simulink model "ACC_speed_change_curve_cs"  (R2016a)
settings: Solver=ode5  SolverMode=SingleTasking  StartTime=0.0  StopTime=inf  FixedStep=1/1000  RelTol=1e-3
PreLoadFcn:
  | mbxruntime.callbacks.PreLoadFcn(bdroot);
  | check_NUTS_defined;
  | 
  | assignin('base',['model_closed_' bdroot],false);addpath('../includes_ACC');
PostLoadFcn:
  | mbxruntime.callbacks.PostLoadFcn(bdroot);
InitFcn:
  | mbxruntime.callbacks.InitFcn(bdroot);
StartFcn:
  | mbxruntime.callbacks.StartFcn(bdroot);
StopFcn:
  | mbxruntime.callbacks.StopFcn(bdroot);
model workspace (MAT data in the model file):
  mbox_table : struct (value not decoded)
  model_closed = 0
  sim_status = 0
undefined symbols (not defined in the file or in its folder): DiscIntNeverNeededParam
undefined symbols (not defined in the file): SteeringColumn, SteeringWheel, WheelL0, WheelL1, WheelR0, WheelR1
libraries: simulink_extras x49, simulink x29, PreScanSimulinkLibrary x24, PreScanUsefulBlocks x2, Solver_SF x1, simulink_need_slupdate x1
(part 15 of 17)

== system ACC_speed_change_curve_cs/Audi_A8_1/ACC_System/TIS2 Straight Road/TIS2 Lead Car Longitudinal Velocity ==
  note: === TIS2 Lead Car Longitudinal Velocity block ===
      |
      |  - computes the leading car absolute velocity and safe distance between the EGO and leading car.
  HWT_dem (s) : Inport
  TIS2 Rangedot [m/s] : Inport  Port=2
  EGO Velocity [m/s] : Inport  Port=3
  Standstill [m] : Inport  Port=4
  Abs : Abs
  Add : Sum  Inputs=+-
  Constant : Constant  Value=0
  Divide : Product  Inputs=*/
  HWT_dem (s)1 : InportShadow
  Product : Product  RndMeth=Zero
  Relational Operator : RelationalOperator  Operator=<=  OutDataTypeStr=boolean
  Switch : Switch  Criteria=u2 > Threshold
  Switch1 : Switch  Criteria=u2 ~= 0
  TIS2 Rangedot [m/s]1 : InportShadow  Port=2
  Safe distance [m] : Outport
  Lead velocity [m/s] : Outport  Port=2
  wires:
  Relational Operator/1 -> Switch/2
  Divide/1 -> Relational Operator/2
  HWT_dem (s)1/1 -> Divide/2
  Standstill [m]/1 -> Switch/1, Divide/1
  Switch/1 -> Safe distance [m]/1
  Product/1 -> Switch/3
  HWT_dem (s)/1 -> Product/2
  Add/1 -> Abs/1
  TIS2 Rangedot [m/s]/1 -> Add/2
  EGO Velocity [m/s]/1 -> Add/1
  Constant/1 -> Switch1/3
  Switch1/1 -> Lead velocity [m/s]/1
  TIS2 Rangedot [m/s]1/1 -> Switch1/2
  Abs/1 -> Product/1, Relational Operator/1, Switch1/1

== system ACC_speed_change_curve_cs/Audi_A8_1/ACC_System/TIS2 Straight Road/TIS2 Objects On Lane ==
  note: === TIS2 Objects On Lane block ===
      |
      |  - decides which objects are on the same lane as the EGO car,
      |    when the EGO car drives straight.
  TIS2_range [m] : Inport
  TIS2_rangedot [m/s] : Inport  Port=2
  TIS2_theta [rad] : Inport  Port=3
  Abs : Abs
  Compare To Constant : simulink/Logic and Bit Operations/Compare To Constant  relop=<  const=LaneWidth/2  OutDataTypeStr=boolean
  Constant : Constant  Value=0
  Product : Product  RndMeth=Zero
  Product1 : Product  RndMeth=Zero
  Switch1 : Switch  Criteria=u2 > Threshold  Threshold=0.5
  Switch3 : Switch  Criteria=u2 > Threshold  Threshold=0.5
  TIS2 range max (higher value) : Constant  Value=5*TISMaxRange(2)
  Trigonometric Function : Trigonometry
  Trigonometric Function1 : Trigonometry  Operator=cos
  TIS2_RANGEDOT [m/s] : Outport
  TIS2_Distance [m] : Outport  Port=2
  wires:
  Compare To Constant/1 -> Switch1/2, Switch3/2
  Constant/1 -> Switch1/3
  TIS2 range max (higher value)/1 -> Switch3/3
  Product1/1 -> Switch3/1
  Trigonometric Function1/1 -> Product1/2
  Abs/1 -> Trigonometric Function/1
  Switch3/1 -> TIS2_Distance [m]/1
  Switch1/1 -> TIS2_RANGEDOT [m/s]/1
  TIS2_rangedot [m/s]/1 -> Switch1/1
  TIS2_range [m]/1 -> Product/1, Product1/1
  Product/1 -> Compare To Constant/1
  Trigonometric Function/1 -> Product/2
  TIS2_theta [rad]/1 -> Trigonometric Function1/1, Abs/1

== system ACC_speed_change_curve_cs/Audi_A8_1/ACC_System/TIS2 Straight Road/TIS2 Sorting Fun ==
  note: === TIS2 Sorting Fun block ===
      |
      |  - transforms information from the second sensor
      |    to the more appropriate form.
  TIS2range [m] : Inport
  TIS2rangedot [m/s] : Inport  Port=2
  TIS2theta [deg] : Inport  Port=3
  Degrees to Radians : simulink_extras/Transformations/Degrees to Radians
  Switch : Switch  Criteria=u2 ~= 0
  Unary Minus : UnaryMinus
  Unary Minus1 : UnaryMinus
  range max (higher value which will not generate high level of HWT flag) : Constant  Value=5*TISMaxRange(2)
  TIS2_RANGE [m] : Outport
  TIS2_RANGEDOT [m/s] : Outport  Port=2
  TIS2_THETA [rad] : Outport  Port=3
  wires:
  Unary Minus1/1 -> TIS2_RANGEDOT [m/s]/1
  TIS2theta [deg]/1 -> Unary Minus/1
  TIS2range [m]/1 -> Switch/2, Switch/1
  Degrees to Radians/1 -> TIS2_THETA [rad]/1
  range max (higher value which will not generate high level of HWT flag)/1 -> Switch/3
  TIS2rangedot [m/s]/1 -> Unary Minus1/1
  Switch/1 -> TIS2_RANGE [m]/1
  Unary Minus/1 -> Degrees to Radians/1

== system ACC_speed_change_curve_cs/Audi_A8_1/ACC_System3/Display/If Action Subsystem ==
  note: === Display Module ===
      |
      |  - calls a GUI, which is updated at each step time,
      |  - Inputs for 'DISPLAY' block (msfcn_PlotSpeed):
      |    1 - RPM
      |    2 - EGO Velocity [kph]
      |    3 - Brake Pressure [bar]
      |    4 - Throttle [%]
      |    5 - ACC Flag
      |    6 - HWT converted
      |    7 - Lead car velocity [m/s]
      |
      |  - Output from DISPLAY block (msfcn_ACC_PlotSpeed function):
      |    1 - ACC system manual switch {0 - system off, 1 - system on}
  RPM1 : Inport
  EGO Velocity [m/s]1 : Inport  Port=2
  Brake_Pressure_[bar]1 : Inport  Port=3
  HWT_%1 : Inport  Port=4
  ACC_flag1 : Inport  Port=5
  Lead_car_velocity_[m/s]1 : Inport  Port=6
  Throttle_[%]1 : Inport  Port=7
  Action Port : ActionPort  PropagateVarSize=During execution  ActionType=then
  Brake Pressure [bar] : Gain  Gain=100/BrakePressureMax
  Brake Pressure [bar]1 : Gain  Gain=3.6
  DISPLAY : M-S-Function  FunctionName=msfcn_ACC_PlotSpeed  Parameters=DisplayFreq DisplaySwitch
      mask Display:
      | port_label('input',1,'RPM');
      | port_label('input',2,'EGO Velocity [km/h]');
      | port_label('input',3,'Brake Pressure [bar]');
      | port_label('input',4,'Throttle [%]');
      | port_label('input',5,'ACC Flag');
      | port_label('input',6,'HWT/HWT_dem-1 [%]');
      | port_label('input',7,'Lead car velocity [m/s]');
      | 
      | port_label('output',1,'System On/Off');
  Gain : Gain  OutDataTypeStr=double
  Rounding Function{,1..4,6} (6 alike) : Rounding  Operator=round
  m/s_kph1 : Gain  Gain=3.6
  "GUI_System ON {1} / OFF {0}1" : Outport  InitialOutput=1
  wires:
  Brake Pressure [bar]1/1 -> Rounding Function1/1
  HWT_%1/1 -> DISPLAY/6
  DISPLAY/1 -> "GUI_System ON {1} / OFF {0}1"/1
  Lead_car_velocity_[m/s]1/1 -> m/s_kph1/1
  ACC_flag1/1 -> Gain/1
  EGO Velocity [m/s]1/1 -> Brake Pressure [bar]1/1
  Gain/1 -> Rounding Function6/1
  Rounding Function6/1 -> DISPLAY/5
  Rounding Function4/1 -> DISPLAY/7
  m/s_kph1/1 -> Rounding Function4/1
  RPM1/1 -> Rounding Function/1
  Throttle_[%]1/1 -> Rounding Function3/1
  Brake_Pressure_[bar]1/1 -> Brake Pressure [bar]/1
  Brake Pressure [bar]/1 -> Rounding Function2/1
  Rounding Function3/1 -> DISPLAY/4
  Rounding Function2/1 -> DISPLAY/3
  Rounding Function1/1 -> DISPLAY/2
  Rounding Function/1 -> DISPLAY/1

== system ACC_speed_change_curve_cs/Audi_A8_1/ACC_System3/Display/If Action Subsystem1 ==
  Action Port : ActionPort  PropagateVarSize=During execution  ActionType=else
  Constant : Constant
  Out1 : Outport  InitialOutput=1
  wires:
  Constant/1 -> Out1/1

== system ACC_speed_change_curve_cs/Audi_A8_1/ACC_System3/Limitations1/cond ==
  In1 : Inport
  Integer Delay : Delay  DelayLength=1/Tsensor  InputProcessing=Inherited  SampleTime=Tsensor
  Logical Operator2 : Logic  Operator=NOT  AllPortsSameDT=off  OutDataTypeStr=boolean
  Logical Operator3 : Logic  Operator=OR  AllPortsSameDT=off  OutDataTypeStr=boolean
  Out1 : Outport
  wires:
  Logical Operator3/1 -> Out1/1
  In1/1 -> Logical Operator2/1
  Integer Delay/1 -> Logical Operator3/2
  Logical Operator2/1 -> Integer Delay/1, Logical Operator3/1

== system ACC_speed_change_curve_cs/Audi_A8_1/ACC_System3/Limitations2/cond1 ==
  In1 : Inport
  Integer Delay : Delay  DelayLength=1/Tsensor  InputProcessing=Inherited  SampleTime=Tsensor
  Logical Operator3 : Logic  Operator=OR  AllPortsSameDT=off  OutDataTypeStr=boolean
  Out1 : Outport
  wires:
  Logical Operator3/1 -> Out1/1
  In1/1 -> Integer Delay/1, Logical Operator3/1
  Integer Delay/1 -> Logical Operator3/2

== system ACC_speed_change_curve_cs/Audi_A8_1/ACC_System3/Radar/Radar ==
  TIS1 Range : Inport
  TIS1 Theta : Inport  Port=2
  TIS2 Range : Inport  Port=3
  TIS2 Theta : Inport  Port=4
  TIS1_index : Inport  Port=5
  TIS2_index : Inport  Port=6
  TIS1_HWT_% : Inport  Port=7
  TIS2_HWT_% : Inport  Port=8
  System switch : Inport  Port=9
  Enable : EnablePort  PropagateVarSize=During execution
  Level-2 M-file S-Function : M-S-Function  FunctionName=msfcn_ACC_radar_graph  Parameters=RadarFreq TISdet TISMaxRange TISMaxTheta RadarSwitch
  Logical Operator : Logic  AllPortsSameDT=off  OutDataTypeStr=boolean
  Logical Operator1 : Logic  AllPortsSameDT=off  OutDataTypeStr=boolean
  Product1 : Product  RndMeth=Zero
  Product2 : Product  RndMeth=Zero
  wires:
  TIS2_index/1 -> Product2/1
  TIS1_index/1 -> Product1/1
  Product1/1 -> Level-2 M-file S-Function/5
  Product2/1 -> Level-2 M-file S-Function/6
  System switch/1 -> Product1/2, Product2/2, Logical Operator/2, Logical Operator1/2
  Logical Operator1/1 -> Level-2 M-file S-Function/8
  Logical Operator/1 -> Level-2 M-file S-Function/7
  TIS2_HWT_%/1 -> Logical Operator1/1
  TIS1_HWT_%/1 -> Logical Operator/1
  TIS2 Theta/1 -> Level-2 M-file S-Function/4
  TIS2 Range/1 -> Level-2 M-file S-Function/3
  TIS1 Theta/1 -> Level-2 M-file S-Function/2
  TIS1 Range/1 -> Level-2 M-file S-Function/1

== system ACC_speed_change_curve_cs/Audi_A8_1/ACC_System3/TIS1 ACC action/If Action Subsystem ==
  rd : Inport
  e : Inport  Port=2
  Vp : Inport  Port=3
  EGO distance : Inport  Port=4
  HWT dem : Inport  Port=5
  th in : Inport  Port=6
  Action Port : ActionPort  PropagateVarSize=During execution  ActionType=then
  If : If  IfExpression=u1 <= 0  SampleTime=Tsensor
  If Action Subsystem : Subsystem  TreatAsAtomicUnit=on
  If Action Subsystem1 : Subsystem  TreatAsAtomicUnit=on
  Merge : Merge
  Merge1 : Merge
  Rate Limiter : RateLimiter  RisingSlewLimit=BrakeMax*1e3  FallingSlewLimit=-BrakeMax*1e3  SampleTimeMode=inherited
  e1 : InportShadow  Port=2
  th in1 : InportShadow  Port=6
  dec : Outport  InitialOutput=0
  throttle : Outport  Port=2  InitialOutput=0
  wires:
  Rate Limiter/1 -> throttle/1
  th in1/1 -> If Action Subsystem1/6(th_in)
  th in/1 -> If Action Subsystem/2(th_in)
  HWT dem/1 -> If Action Subsystem1/5(HWT_dem)
  EGO distance/1 -> If Action Subsystem1/4(EGO distance)
  e1/1 -> If Action Subsystem1/2(e)
  Vp/1 -> If Action Subsystem1/3(Vp)
  Merge1/1 -> Rate Limiter/1
  Merge/1 -> dec/1
  If Action Subsystem1/2(throttle) -> Merge1/2
  If Action Subsystem/2(throttle) -> Merge1/1
  If Action Subsystem1/1(dec) -> Merge/2
  If Action Subsystem/1(brake) -> Merge/1
  e/1 -> If Action Subsystem/1(e)
  If/2 -> If Action Subsystem1/Action
  If/1 -> If Action Subsystem/Action
  rd/1 -> If Action Subsystem1/1(rd), If/1

== system ACC_speed_change_curve_cs/Audi_A8_1/ACC_System3/TIS1 ACC action/If Action Subsystem1 ==
  rd : Inport
  e : Inport  Port=2
  Vp : Inport  Port=3
  EGO dis : Inport  Port=4
  HWT dem : Inport  Port=5
  Action Port : ActionPort  PropagateVarSize=During execution  ActionType=else
  If : If  IfExpression=u1 <= 0  SampleTime=Tsensor
  If Action Subsystem : Subsystem  TreatAsAtomicUnit=on
  If Action Subsystem1 : Subsystem  TreatAsAtomicUnit=on
  Merge : Merge
  Merge1 : Merge
  dec : Outport  InitialOutput=0
  throttle : Outport  Port=2  InitialOutput=0
  wires:
  HWT dem/1 -> If Action Subsystem1/5(HWT dem)
  EGO dis/1 -> If Action Subsystem1/4(Ego distance)
  e/1 -> If Action Subsystem1/2(e)
  If Action Subsystem/2(throttle) -> Merge1/1
  If Action Subsystem1/1(dec) -> Merge/2
  Merge1/1 -> throttle/1
  Merge/1 -> dec/1
  If Action Subsystem1/2(throttle) -> Merge1/2
  If Action Subsystem/1(dec) -> Merge/1
  Vp/1 -> If Action Subsystem1/3(Vp)
  If/2 -> If Action Subsystem1/Action
  If/1 -> If Action Subsystem/Action
  rd/1 -> If Action Subsystem1/1(rd), If/1

== system ACC_speed_change_curve_cs/Audi_A8_1/ACC_System3/TIS1 Bend Road/Hold ==
  HWTflagIN : Inport
  lead_vel_in : Inport  Port=2
  HWTflagIN1 : InportShadow
  If : If  IfExpression=u1 < 0.1  SampleTime=Tsensor
  If Action Subsystem : Subsystem  TreatAsAtomicUnit=on
  If Action Subsystem1 : Subsystem  TreatAsAtomicUnit=on
  Merge : Merge
  HWT_flag : Outport
  wires:
  HWTflagIN1/1 -> If Action Subsystem/1(In1)
  HWTflagIN/1 -> If Action Subsystem1/1(In1)
  Merge/1 -> HWT_flag/1
  If Action Subsystem1/1(Out1) -> Merge/2
  If Action Subsystem/1(Out1) -> Merge/1
  If/2 -> If Action Subsystem1/Action
  If/1 -> If Action Subsystem/Action
  lead_vel_in/1 -> If/1

== system ACC_speed_change_curve_cs/Audi_A8_1/ACC_System3/TIS1 Bend Road/Lead Car Longitudinal Velocity ==
  note: === TIS1 Lead Car Longitudinal Velocity block ===
      |
      |  - computes the leading car absolute velocity and safe distance between the EGO and leading car.
  HWT_dem (s) : Inport
  TIS1 Rangedot [m/s] : Inport  Port=2
  EGO Velocity [m/s] : Inport  Port=3
  Standstill [m] : Inport  Port=4
  theta [rad] : Inport  Port=5
  lambda [rad] : Inport  Port=6
  TIS1 Range [m] : Inport  Port=7
  Abs : Abs
  Add : Sum  Inputs=+-  RndMeth=Zero
  Add1 : Sum  Inputs=+-
  Constant : Constant  Value=0
  Divide : Product  Inputs=*/
  Divide2 : Product  Inputs=*/
  HWT_dem (s)1 : InportShadow
  Product : Product  RndMeth=Zero
  Relational Operator : RelationalOperator  Operator=<=  OutDataTypeStr=boolean
  Switch : Switch  Criteria=u2 > Threshold
  Switch1 : Switch  Threshold=TISMaxRange(1)
  Trigonometric Function : Trigonometry  Operator=cos
  Safe distance [m] : Outport
  Lead velocity [m/s] : Outport  Port=2
  wires:
  Switch1/1 -> Lead velocity [m/s]/1
  Constant/1 -> Switch1/1
  TIS1 Range [m]/1 -> Switch1/2
  Abs/1 -> Switch1/3, Relational Operator/1, Product/1
  Divide2/1 -> Add/2
  Trigonometric Function/1 -> Divide2/2
  Add1/1 -> Trigonometric Function/1
  theta [rad]/1 -> Add1/2
  lambda [rad]/1 -> Add1/1
  EGO Velocity [m/s]/1 -> Add/1
  TIS1 Rangedot [m/s]/1 -> Divide2/1
  Add/1 -> Abs/1
  HWT_dem (s)/1 -> Product/2
  Product/1 -> Switch/3
  Switch/1 -> Safe distance [m]/1
  Standstill [m]/1 -> Divide/1, Switch/1
  HWT_dem (s)1/1 -> Divide/2
  Divide/1 -> Relational Operator/2
  Relational Operator/1 -> Switch/2

== system ACC_speed_change_curve_cs/Audi_A8_1/ACC_System3/TIS1 Bend Road/TIS1 Closest Object On Bend Road ==
  note: === TIS1 Closest Object block ===
      |
      |  - passing through data about potentially the most dangerous object driving on the bend road.
  index : Inport
  TIS1_range [m] : Inport  Port=2
  TIS1_rangedot [m] : Inport  Port=3
  TIS1_theta [rad] : Inport  Port=4
  TIS1_Distance [m] : Inport  Port=5
  TIS1_lambda [rad] : Inport  Port=6
  Constant2 : Constant  Value=TISMaxRange(1)
  Selector{1..3,6..7} (5 alike) : Selector  InputPortWidth=TISdet(1)  IndexOptions=Index vector (port)  Indices=[1 3]  OutputSizes=1
  Switch : Switch  Criteria=u2 ~= 0
  range [m] : Outport
  rangedot [m/s] : Outport  Port=2
  theta [rad] : Outport  Port=3
  Distance [m] : Outport  Port=4
  lambda [rad] : Outport  Port=5
  wires:
  Switch/1 -> Distance [m]/1
  Constant2/1 -> Switch/3
  Selector6/1 -> Switch/1, Switch/2
  Selector7/1 -> lambda [rad]/1
  Selector3/1 -> theta [rad]/1
  Selector2/1 -> rangedot [m/s]/1
  Selector1/1 -> range [m]/1
  TIS1_lambda [rad]/1 -> Selector7/1
  TIS1_Distance [m]/1 -> Selector6/1
  TIS1_theta [rad]/1 -> Selector3/1
  index/1 -> Selector7/2, Selector6/2, Selector3/2, Selector2/2, Selector1/2
  TIS1_range [m]/1 -> Selector1/1
  TIS1_rangedot [m]/1 -> Selector2/1

== system ACC_speed_change_curve_cs/Audi_A8_1/ACC_System3/TIS1 Bend Road/TIS1 HWT Computing ==
  note: === TIS1 HWT Computing block===
      |
      |  - computes HeadWay Time (HWT) as it is defined in ISO norms.
  Distance [m] : Inport
  Velocity [m/s] : Inport  Port=2
  If : If
  If Action Subsystem : Subsystem  TreatAsAtomicUnit=on
  If Action Subsystem1 : Subsystem  TreatAsAtomicUnit=on
  Merge : Merge
  HWT [s] : Outport
  wires:
  Distance [m]/1 -> If Action Subsystem/1(Distance [m])
  Merge/1 -> HWT [s]/1
  If Action Subsystem1/1(Out1) -> Merge/2
  If Action Subsystem/1(HWT [s]) -> Merge/1
  If/2 -> If Action Subsystem1/Action
  If/1 -> If Action Subsystem/Action
  Velocity [m/s]/1 -> If Action Subsystem/2(Velocity [m/s]), If/1

== system ACC_speed_change_curve_cs/Audi_A8_1/ACC_System3/TIS1 Bend Road/TIS1 HWT Flag ==
  note: === TIS1 HWT Flag block ===
      |
      |  - outputs the HeadWay Time (HWT) flag,
      |  - holds a high level if the criteria were met,
      |  - sets HWT flag to low level if leading car
      |    went outside the scope of the sensors.
  Distance closest [m] : Inport
  HWT [s] : Inport  Port=2
  HWT_dem [s] : Inport  Port=3
  Standstill distance : Inport  Port=4
  Abs : Abs
  Compare To Constant1 : simulink/Logic and Bit Operations/Compare To Constant  relop===  const=TISMaxRange(1)  OutDataTypeStr=uint8
  Constant : Constant
  Constant1 : Constant  Value=0
  Data Type Conversion : DataTypeConversion
  Data Type Conversion1 : DataTypeConversion
  Discrete-Time Integrator : DiscreteIntegrator  ExternalReset=level  SampleTime=Tsensor  ICPrevOutput=DiscIntNeverNeededParam  ICPrevScaledInput=DiscIntNeverNeededParam
  Distance closest [m]1 : InportShadow
  Gain : Gain  Gain=2
  Gain1 : Gain
  Gain2 : Gain  Gain=1e6  OutDataTypeStr=double
  Gain3 : Gain  Gain=1e6  OutDataTypeStr=double
  Gain4 : Gain  Gain=1.25
  Gain6 : Gain  Gain=100
  Gain7 : Gain  Gain=1.25
  Gain8 : Gain  Gain=0.01
  HWT [s]1 : InportShadow  Port=2
  HWT [s]2 : InportShadow  Port=2
  HWT_dem [s]1 : InportShadow  Port=3
  HWT_dem [s]2 : InportShadow  Port=3
  Logical Operator : Logic  AllPortsSameDT=off  OutDataTypeStr=boolean
  Logical Operator1 : Logic  AllPortsSameDT=off  OutDataTypeStr=boolean
  Logical Operator2 : Logic  Operator=OR  Inputs=3  AllPortsSameDT=off  OutDataTypeStr=boolean
  Logical Operator3 : Logic  AllPortsSameDT=off  OutDataTypeStr=boolean
  MinMax : MinMax
  MinMax2 : MinMax
  Relational Operator : RelationalOperator  Operator=<=  OutDataTypeStr=boolean
  Relational Operator1 : RelationalOperator  OutDataTypeStr=boolean
  Relational Operator2 : RelationalOperator  Operator=>  OutDataTypeStr=boolean
  Relational Operator4 : RelationalOperator  Operator=>  OutDataTypeStr=boolean
  Rounding Function : Rounding
  Sum of Elements : Sum  Inputs=+
  Switch : Switch  Criteria=u2 > Threshold
  HWT_flag : Outport
  wires:
  Data Type Conversion1/1 -> Gain3/1
  Data Type Conversion/1 -> Gain2/1
  Gain7/1 -> Relational Operator4/2
  Gain8/1 -> Relational Operator4/1
  MinMax2/1 -> Gain6/1
  Rounding Function/1 -> Gain8/1
  Gain6/1 -> Rounding Function/1
  HWT [s]2/1 -> MinMax2/1
  HWT_dem [s]2/1 -> Gain7/1
  Relational Operator4/1 -> Logical Operator2/3
  Gain4/1 -> Relational Operator/2
  Switch/1 -> HWT_flag/1
  Constant1/1 -> Switch/3
  Constant/1 -> Switch/1
  Abs/1 -> Switch/2
  Discrete-Time Integrator/1 -> Abs/1
  Gain3/1 -> Discrete-Time Integrator/1
  Gain2/1 -> Discrete-Time Integrator/2
  Logical Operator3/1 -> Logical Operator2/2
  MinMax/1 -> Logical Operator3/1
  Relational Operator2/1 -> Logical Operator3/2
  Standstill distance/1 -> Relational Operator2/2
  Distance closest [m]1/1 -> Relational Operator2/1
  HWT_dem [s]1/1 -> Gain/1
  Logical Operator2/1 -> Data Type Conversion/1
  Gain1/1 -> MinMax/1
  Relational Operator1/1 -> Gain1/1
  Gain/1 -> Relational Operator1/2
  HWT [s]1/1 -> Relational Operator1/1
  Compare To Constant1/1 -> Logical Operator1/1, Logical Operator1/2
  HWT [s]/1 -> Relational Operator/1
  HWT_dem [s]/1 -> Gain4/1
  Relational Operator/1 -> Sum of Elements/1
  Sum of Elements/1 -> Logical Operator/1, Logical Operator/2
  Logical Operator/1 -> Data Type Conversion1/1
  Distance closest [m]/1 -> Compare To Constant1/1
  Logical Operator1/1 -> Logical Operator2/1

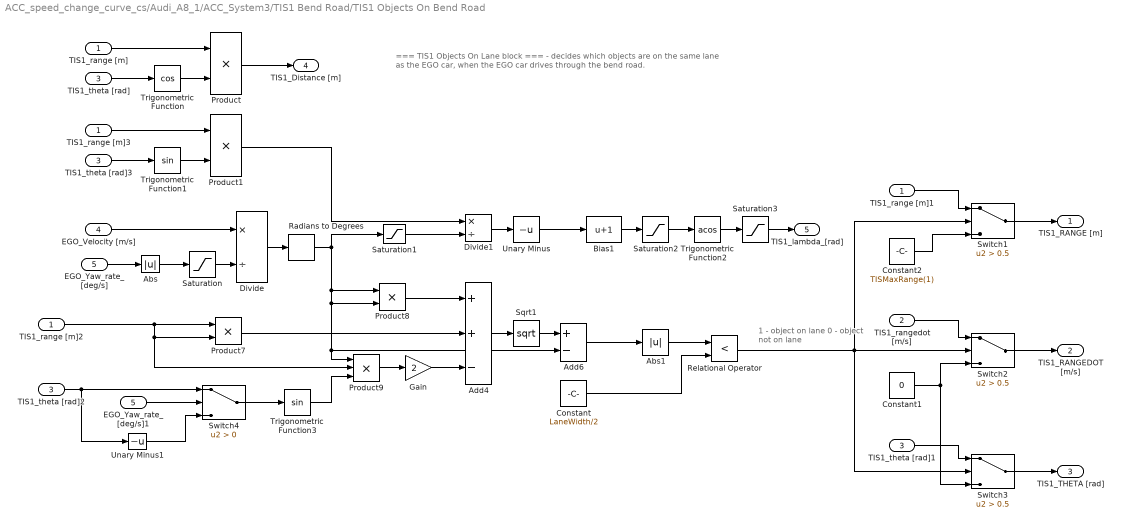
== system ACC_speed_change_curve_cs/Audi_A8_1/ACC_System3/TIS1 Bend Road/TIS1 Objects On Bend Road ==
  note: === TIS1 Objects On Lane block ===
      |
      |  - decides which objects are on the same lane as the EGO car,
      |     when the EGO car drives through the bend road.
  note: 1  - object      on lane
      | 0 - object not on lane
  TIS1_range [m] : Inport
  TIS1_rangedot [m/s] : Inport  Port=2
  TIS1_theta [rad] : Inport  Port=3
  EGO_Velocity [m/s] : Inport  Port=4
  EGO_Yaw_rate_[deg/s] : Inport  Port=5
  Abs : Abs
  Abs1 : Abs
  Add4 : Sum  Inputs=++-
  Add6 : Sum  Inputs=+-
  Bias1 : Bias  Bias=1
  Constant : Constant  Value=LaneWidth/2
  Constant1 : Constant  Value=0
  Constant2 : Constant  Value=TISMaxRange(1)
  Divide : Product  Inputs=*/
  Divide1 : Product  Inputs=*/
  EGO_Yaw_rate_[deg/s]1 : InportShadow  Port=5
  Gain : Gain  Gain=2
  Product{,1,7..8} (4 alike) : Product  RndMeth=Zero
  Product9 : Product  Inputs=3  RndMeth=Zero
  Radians to Degrees : simulink_extras/Transformations/Radians to Degrees
  Relational Operator : RelationalOperator  Operator=<  OutDataTypeStr=boolean
  Saturation : Saturate  UpperLimit=inf  LowerLimit=1e-6
  Saturation1 : Saturate  UpperLimit=inf  LowerLimit=1e-6
  Saturation2 : Saturate  UpperLimit=1  LowerLimit=-1
  Saturation3 : Saturate  UpperLimit=pi  LowerLimit=0
  Sqrt1 : Math  Operator=sqrt  SaturateOnIntegerOverflow=on
  Switch1 : Switch  Criteria=u2 > Threshold  Threshold=0.5
  Switch2 : Switch  Criteria=u2 > Threshold  Threshold=0.5
  Switch3 : Switch  Criteria=u2 > Threshold  Threshold=0.5
  Switch4 : Switch  Criteria=u2 > Threshold
  TIS1_range [m]1 : InportShadow
  TIS1_range [m]2 : InportShadow
  TIS1_range [m]3 : InportShadow
  TIS1_theta [rad]1 : InportShadow  Port=3
  TIS1_theta [rad]2 : InportShadow  Port=3
  TIS1_theta [rad]3 : InportShadow  Port=3
  Trigonometric Function : Trigonometry  Operator=cos
  Trigonometric Function1 : Trigonometry
  Trigonometric Function2 : Trigonometry  Operator=acos
  Trigonometric Function3 : Trigonometry
  Unary Minus : UnaryMinus
  Unary Minus1 : UnaryMinus
  TIS1_RANGE [m] : Outport
  TIS1_RANGEDOT [m/s] : Outport  Port=2
  TIS1_THETA [rad] : Outport  Port=3
  TIS1_Distance [m] : Outport  Port=4
  TIS1_lambda_[rad] : Outport  Port=5
  wires:
  Abs/1 -> Saturation/1
  Saturation3/1 -> TIS1_lambda_[rad]/1
  Saturation2/1 -> Trigonometric Function2/1
  Saturation1/1 -> Divide1/2
  Saturation/1 -> Divide/2
  Constant/1 -> Relational Operator/2
  Abs1/1 -> Relational Operator/1
  Product1/1 -> Divide1/1
  TIS1_theta [rad]3/1 -> Trigonometric Function1/1
  TIS1_range [m]3/1 -> Product1/1
  TIS1_range [m]2/1 -> Product9/2, Product7/2, Product7/1
  Unary Minus1/1 -> Switch4/3
  TIS1_theta [rad]2/1 -> Unary Minus1/1, Switch4/1
  Switch4/1 -> Trigonometric Function3/1
  EGO_Yaw_rate_[deg/s]1/1 -> Switch4/2
  Add6/1 -> Abs1/1
  Sqrt1/1 -> Add6/1
  Add4/1 -> Sqrt1/1
  Trigonometric Function3/1 -> Product9/3
  Product9/1 -> Gain/1
  Gain/1 -> Add4/3
  Product7/1 -> Add4/2
  Product8/1 -> Add4/1
  Product/1 -> TIS1_Distance [m]/1
  Trigonometric Function2/1 -> Saturation3/1
  Unary Minus/1 -> Bias1/1
  Divide1/1 -> Unary Minus/1
  Bias1/1 -> Saturation2/1
  Switch3/1 -> TIS1_THETA [rad]/1
  Switch2/1 -> TIS1_RANGEDOT [m/s]/1
  Switch1/1 -> TIS1_RANGE [m]/1
  Constant2/1 -> Switch1/3
  Constant1/1 -> Switch3/3, Switch2/3
  TIS1_theta [rad]1/1 -> Switch3/1
  TIS1_range [m]1/1 -> Switch1/1
  TIS1_rangedot [m/s]/1 -> Switch2/1
  Relational Operator/1 -> Switch3/2, Switch2/2, Switch1/2
  Radians to Degrees/1 -> Saturation1/1, Add6/2, Product9/1, Product8/2, Product8/1
  Divide/1 -> Radians to Degrees/1
  EGO_Yaw_rate_[deg/s]/1 -> Abs/1
  EGO_Velocity [m/s]/1 -> Divide/1
  Trigonometric Function1/1 -> Product1/2
  Trigonometric Function/1 -> Product/2
  TIS1_theta [rad]/1 -> Trigonometric Function/1
  TIS1_range [m]/1 -> Product/1

== system ACC_speed_change_curve_cs/Audi_A8_1/ACC_System3/TIS1 Bend Road/TIS1 Sorting  Fun ==
  note: === TIS1 Sorting Fun block ===
      |
      |  - transforms information from the first sensor
      |    to the more appropriate form.
  TIS1range [m] : Inport
  TIS1rangedot [m/s] : Inport  Port=2
  TIS1theta [deg] : Inport  Port=3
  Degrees to Radians : simulink_extras/Transformations/Degrees to Radians
  Switch : Switch  Criteria=u2 ~= 0
  Unary Minus : UnaryMinus
  Unary Minus1 : UnaryMinus
  range max : Constant  Value=TISMaxRange(1)
  TIS1_RANGE [m] : Outport
  TIS1_RANGEDOT [m/s] : Outport  Port=2
  TIS1_THETA [rad] : Outport  Port=3
  wires:
  Unary Minus/1 -> Degrees to Radians/1
  Switch/1 -> TIS1_RANGE [m]/1
  TIS1rangedot [m/s]/1 -> Unary Minus1/1
  range max/1 -> Switch/3
  Degrees to Radians/1 -> TIS1_THETA [rad]/1
  TIS1range [m]/1 -> Switch/1, Switch/2
  TIS1theta [deg]/1 -> Unary Minus/1
  Unary Minus1/1 -> TIS1_RANGEDOT [m/s]/1

== system ACC_speed_change_curve_cs/Audi_A8_1/ACC_System3/TIS1 Straight Road/Hold ==
  HWTflagIN : Inport
  lead_vel_in : Inport  Port=2
  HWTflagIN1 : InportShadow
  If : If  IfExpression=u1 < 0.1  SampleTime=Tsensor
  If Action Subsystem : Subsystem  TreatAsAtomicUnit=on
  If Action Subsystem1 : Subsystem  TreatAsAtomicUnit=on
  Merge : Merge
  HWT_flag : Outport
  wires:
  HWTflagIN1/1 -> If Action Subsystem/1(In1)
  HWTflagIN/1 -> If Action Subsystem1/1(In1)
  Merge/1 -> HWT_flag/1
  If Action Subsystem1/1(Out1) -> Merge/2
  If Action Subsystem/1(Out1) -> Merge/1
  If/2 -> If Action Subsystem1/Action
  If/1 -> If Action Subsystem/Action
  lead_vel_in/1 -> If/1

== system ACC_speed_change_curve_cs/Audi_A8_1/ACC_System3/TIS1 Straight Road/TIS1 Closest Object ==
  note: === TIS1 Closest Object block ===
      |
      |  - passing through data about potentially the most dangerous object driving on the straight road.
  TIS1_rangedot [m/s] : Inport
  TIS1_Distance [m] : Inport  Port=2
  index : Inport  Port=3
  Selector1 : Selector  InputPortWidth=TISdet(1)  IndexOptions=Index vector (port)  Indices=[1 3]  OutputSizes=1
  Selector2 : Selector  InputPortWidth=TISdet(1)  IndexOptions=Index vector (port)  Indices=[1 3]  OutputSizes=1
  rangedot [m/s] : Outport
  Distance [m/s] : Outport  Port=2
  wires:
  Selector2/1 -> Distance [m/s]/1
  TIS1_Distance [m]/1 -> Selector2/1
  Selector1/1 -> rangedot [m/s]/1
  TIS1_rangedot [m/s]/1 -> Selector1/1
  index/1 -> Selector2/2, Selector1/2

== system ACC_speed_change_curve_cs/Audi_A8_1/ACC_System3/TIS1 Straight Road/TIS1 HWT Computing ==
  note: === TIS1 HWT Computing block===
      |
      |  - computes HeadWay Time (HWT) as it is defined in ISO norms.
  Distance [m] : Inport
  HWT demanded : Inport  Port=2
  Velocity [m/s] : Inport  Port=3
  If : If
  If Action Subsystem : Subsystem  TreatAsAtomicUnit=on
  If Action Subsystem1 : Subsystem  TreatAsAtomicUnit=on
  Merge : Merge
  HWT [s] : Outport
  wires:
  HWT demanded/1 -> If Action Subsystem1/1(HWT demanded [s])
  Distance [m]/1 -> If Action Subsystem/1(Distance [m])
  Merge/1 -> HWT [s]/1
  If Action Subsystem1/1(Out1) -> Merge/2
  If Action Subsystem/1(HWT [s]) -> Merge/1
  If/2 -> If Action Subsystem1/Action
  If/1 -> If Action Subsystem/Action
  Velocity [m/s]/1 -> If Action Subsystem/2(Velocity [m/s]), If/1

== system ACC_speed_change_curve_cs/Audi_A8_1/ACC_System3/TIS1 Straight Road/TIS1 HWT Computing1 ==
  note: === TIS1 HWT Computing block===
      |
      |  - computes HeadWay Time (HWT) as it is defined in ISO norms.
  Distance [m] : Inport
  Velocity [m/s] : Inport  Port=2
  If : If
  If Action Subsystem : Subsystem  TreatAsAtomicUnit=on
  If Action Subsystem1 : Subsystem  TreatAsAtomicUnit=on
  Merge : Merge
  HWT [s] : Outport
  wires:
  Distance [m]/1 -> If Action Subsystem/1(Distance [m])
  Merge/1 -> HWT [s]/1
  If Action Subsystem1/1(Out1) -> Merge/2
  If Action Subsystem/1(HWT [s]) -> Merge/1
  If/2 -> If Action Subsystem1/Action
  If/1 -> If Action Subsystem/Action
  Velocity [m/s]/1 -> If Action Subsystem/2(Velocity [m/s]), If/1

== system ACC_speed_change_curve_cs/Audi_A8_1/ACC_System3/TIS1 Straight Road/TIS1 HWT Flag ==
  note: === TIS1 HWT Flag block ===
      |
      |  - outputs the HeadWay Time (HWT) flag,
      |  - holds a high level if the criteria were met,
      |  - sets HWT flag to low level if leading car
      |    went outside the scope of the sensors.
  Distance closest [m] : Inport
  HWT_dem [s] : Inport  Port=2
  HWT [s] : Inport  Port=3
  Standstill distance : Inport  Port=4
  Abs : Abs
  Compare To Constant1 : simulink/Logic and Bit Operations/Compare To Constant  relop===  const=TISMaxRange(1)  OutDataTypeStr=uint8
  Constant : Constant
  Constant1 : Constant  Value=0
  Data Type Conversion : DataTypeConversion
  Data Type Conversion1 : DataTypeConversion
  Discrete-Time Integrator : DiscreteIntegrator  ExternalReset=level  SampleTime=Tsensor  ICPrevOutput=DiscIntNeverNeededParam  ICPrevScaledInput=DiscIntNeverNeededParam
  Distance closest [m]1 : InportShadow
  Gain : Gain  Gain=2
  Gain1 : Gain
  Gain2 : Gain  Gain=1e6  OutDataTypeStr=double
  Gain3 : Gain  Gain=1e6  OutDataTypeStr=double
  Gain4 : Gain  Gain=1.25
  Gain6 : Gain  Gain=100
  Gain7 : Gain  Gain=1.25
  Gain8 : Gain  Gain=0.01
  HWT [s]1 : InportShadow  Port=3
  HWT [s]3 : InportShadow  Port=3
  HWT_dem [s]1 : InportShadow  Port=2
  HWT_dem [s]2 : InportShadow  Port=2
  Logical Operator : Logic  AllPortsSameDT=off  OutDataTypeStr=boolean
  Logical Operator1 : Logic  AllPortsSameDT=off  OutDataTypeStr=boolean
  Logical Operator2 : Logic  Operator=OR  Inputs=3  AllPortsSameDT=off  OutDataTypeStr=boolean
  Logical Operator3 : Logic  AllPortsSameDT=off  OutDataTypeStr=boolean
  MinMax : MinMax
  MinMax2 : MinMax
  Relational Operator : RelationalOperator  Operator=<=  OutDataTypeStr=boolean
  Relational Operator1 : RelationalOperator  OutDataTypeStr=boolean
  Relational Operator2 : RelationalOperator  Operator=>  OutDataTypeStr=boolean
  Relational Operator4 : RelationalOperator  Operator=>  OutDataTypeStr=boolean
  Rounding Function : Rounding
  Sum of Elements : Sum  Inputs=+
  Switch : Switch  Criteria=u2 > Threshold
  HWT_flag : Outport
  wires:
  Data Type Conversion1/1 -> Gain3/1
  Data Type Conversion/1 -> Gain2/1
  Relational Operator4/1 -> Logical Operator2/3
  Gain7/1 -> Relational Operator4/2
  Gain8/1 -> Relational Operator4/1
  MinMax2/1 -> Gain6/1
  Rounding Function/1 -> Gain8/1
  Gain6/1 -> Rounding Function/1
  HWT [s]3/1 -> MinMax2/1
  HWT_dem [s]2/1 -> Gain7/1
  Gain4/1 -> Relational Operator/2
  Constant1/1 -> Switch/3
  Constant/1 -> Switch/1
  Abs/1 -> Switch/2
  Switch/1 -> HWT_flag/1
  Discrete-Time Integrator/1 -> Abs/1
  Gain3/1 -> Discrete-Time Integrator/1
  Gain2/1 -> Discrete-Time Integrator/2
  Logical Operator3/1 -> Logical Operator2/2
  MinMax/1 -> Logical Operator3/1
  Relational Operator2/1 -> Logical Operator3/2
  Standstill distance/1 -> Relational Operator2/2
  Distance closest [m]1/1 -> Relational Operator2/1
  HWT_dem [s]1/1 -> Gain/1
  Logical Operator2/1 -> Data Type Conversion/1
  Gain1/1 -> MinMax/1
  Relational Operator1/1 -> Gain1/1
  Gain/1 -> Relational Operator1/2
  HWT [s]1/1 -> Relational Operator1/1
  Compare To Constant1/1 -> Logical Operator1/1, Logical Operator1/2
  HWT [s]/1 -> Relational Operator/1
  HWT_dem [s]/1 -> Gain4/1
  Relational Operator/1 -> Sum of Elements/1
  Sum of Elements/1 -> Logical Operator/1, Logical Operator/2
  Logical Operator/1 -> Data Type Conversion1/1
  Distance closest [m]/1 -> Compare To Constant1/1
  Logical Operator1/1 -> Logical Operator2/1

== system ACC_speed_change_curve_cs/Audi_A8_1/ACC_System3/TIS1 Straight Road/TIS1 Lead Car Longitudinal Velocity ==
  note: === TIS1 Lead Car Longitudinal Velocity block ===
      |
      |  - computes the leading car absolute velocity and safe distance between the EGO and leading car.
  HWT_dem (s) : Inport
  TIS1 Rangedot [m/s] : Inport  Port=2
  EGO Velocity [m/s] : Inport  Port=3
  Standstill [m] : Inport  Port=4
  Abs : Abs
  Add : Sum  Inputs=+-
  Constant : Constant  Value=0
  Divide : Product  Inputs=*/
  HWT_dem (s)1 : InportShadow
  Product : Product  RndMeth=Zero
  Relational Operator : RelationalOperator  Operator=<=  OutDataTypeStr=boolean
  Switch : Switch  Criteria=u2 > Threshold
  Switch1 : Switch  Criteria=u2 ~= 0
  TIS1 Rangedot [m/s]1 : InportShadow  Port=2
  lead_velocity [m/s] : Outport
  Safe distance [m] : Outport  Port=2
  wires:
  Abs/1 -> Switch1/1, Relational Operator/1, Product/1
  Switch1/1 -> lead_velocity [m/s]/1
  Constant/1 -> Switch1/3
  TIS1 Rangedot [m/s]1/1 -> Switch1/2
  Relational Operator/1 -> Switch/2
  Divide/1 -> Relational Operator/2
  HWT_dem (s)1/1 -> Divide/2
  Standstill [m]/1 -> Switch/1, Divide/1
  Switch/1 -> Safe distance [m]/1
  Product/1 -> Switch/3
  HWT_dem (s)/1 -> Product/2
  Add/1 -> Abs/1
  TIS1 Rangedot [m/s]/1 -> Add/2
  EGO Velocity [m/s]/1 -> Add/1

== system ACC_speed_change_curve_cs/Audi_A8_1/ACC_System3/TIS1 Straight Road/TIS1 Objects On Lane ==
  note: === TIS1 Objects On Lane block ===
      |
      |  - decides which objects are on the same lane as the EGO car,
      |    when the EGO car drives straight.
  TIS1_range [m] : Inport
  TIS1_rangedot [m/s] : Inport  Port=2
  TIS1_theta [rad] : Inport  Port=3
  Abs : Abs
  Compare To Constant : simulink/Logic and Bit Operations/Compare To Constant  relop=<  const=LaneWidth/2  OutDataTypeStr=boolean
  Constant : Constant  Value=0
  Product : Product  RndMeth=Zero
  Product1 : Product  RndMeth=Zero
  Switch1 : Switch  Criteria=u2 > Threshold  Threshold=0.5
  Switch3 : Switch  Criteria=u2 > Threshold  Threshold=0.5
  TIS1 range max : Constant  Value=TISMaxRange(1)
  Trigonometric Function : Trigonometry
  Trigonometric Function1 : Trigonometry  Operator=cos
  TIS1_RANGEDOT [m/s] : Outport
  TIS1_Distance [m] : Outport  Port=2
  wires:
  Compare To Constant/1 -> Switch3/2, Switch1/2
  Constant/1 -> Switch1/3
  TIS1 range max/1 -> Switch3/3
  Product1/1 -> Switch3/1
  Trigonometric Function1/1 -> Product1/2
  Abs/1 -> Trigonometric Function/1
  Switch3/1 -> TIS1_Distance [m]/1
  Switch1/1 -> TIS1_RANGEDOT [m/s]/1
  TIS1_rangedot [m/s]/1 -> Switch1/1
  TIS1_range [m]/1 -> Product1/1, Product/1
  Product/1 -> Compare To Constant/1
  Trigonometric Function/1 -> Product/2
  TIS1_theta [rad]/1 -> Trigonometric Function1/1, Abs/1

== system ACC_speed_change_curve_cs/Audi_A8_1/ACC_System3/TIS1 Straight Road/TIS1 Sorting Fun ==
  note: === TIS1 Sorting Fun block ===
      |
      |  - transforms information from the first sensor
      |    to the more appropriate form.
  TIS1range [m] : Inport
  TIS1rangedot [m/s] : Inport  Port=2
  TIS1theta [deg] : Inport  Port=3
  Degrees to Radians : simulink_extras/Transformations/Degrees to Radians
  Switch : Switch  Criteria=u2 ~= 0
  Unary Minus : UnaryMinus
  Unary Minus1 : UnaryMinus
  range max : Constant  Value=TISMaxRange(1)
  TIS1_RANGE [m] : Outport
  TIS1_RANGEDOT [m/s] : Outport  Port=2
  TIS1_THETA [rad] : Outport  Port=3
  wires:
  Unary Minus1/1 -> TIS1_RANGEDOT [m/s]/1
  TIS1theta [deg]/1 -> Unary Minus/1
  TIS1range [m]/1 -> Switch/1, Switch/2
  Degrees to Radians/1 -> TIS1_THETA [rad]/1
  range max/1 -> Switch/3
  TIS1rangedot [m/s]/1 -> Unary Minus1/1
  Switch/1 -> TIS1_RANGE [m]/1
  Unary Minus/1 -> Degrees to Radians/1

== system ACC_speed_change_curve_cs/Audi_A8_1/ACC_System3/TIS2 ACC action/If Action Subsystem ==
  rd : Inport
  e : Inport  Port=2
  Vp : Inport  Port=3
  EGO distance : Inport  Port=4
  HWT dem : Inport  Port=5
  th in : Inport  Port=6
  Action Port : ActionPort  PropagateVarSize=During execution  ActionType=then
  If : If  IfExpression=u1 <= 0
  If Action Subsystem : Subsystem  TreatAsAtomicUnit=on
  If Action Subsystem1 : Subsystem  TreatAsAtomicUnit=on
  Merge : Merge
  Merge1 : Merge
  e1 : InportShadow  Port=2
  th in1 : InportShadow  Port=6
  dec : Outport  InitialOutput=0
  throttle : Outport  Port=2  InitialOutput=0
  wires:
  th in1/1 -> If Action Subsystem1/6(th_in)
  th in/1 -> If Action Subsystem/2(th_in)
  HWT dem/1 -> If Action Subsystem1/5(HWT_dem)
  EGO distance/1 -> If Action Subsystem1/4(EGO distance)
  e1/1 -> If Action Subsystem1/2(e)
  Vp/1 -> If Action Subsystem1/3(Vp)
  Merge1/1 -> throttle/1
  Merge/1 -> dec/1
  If Action Subsystem1/2(throttle) -> Merge1/2
  If Action Subsystem/2(throttle) -> Merge1/1
  If Action Subsystem1/1(dec) -> Merge/2
  If Action Subsystem/1(brake) -> Merge/1
  e/1 -> If Action Subsystem/1(e)
  If/2 -> If Action Subsystem1/Action
  If/1 -> If Action Subsystem/Action
  rd/1 -> If Action Subsystem1/1(rd), If/1

== system ACC_speed_change_curve_cs/Audi_A8_1/ACC_System3/TIS2 ACC action/If Action Subsystem1 ==
  rd : Inport
  e : Inport  Port=2
  Vp : Inport  Port=3
  EGO dis : Inport  Port=4
  HWT dem : Inport  Port=5
  Action Port : ActionPort  PropagateVarSize=During execution  ActionType=else
  If : If  IfExpression=u1 <= 0
  If Action Subsystem : Subsystem  TreatAsAtomicUnit=on
  If Action Subsystem1 : Subsystem  TreatAsAtomicUnit=on
  Merge : Merge
  Merge1 : Merge
  dec : Outport  InitialOutput=0
  throttle : Outport  Port=2  InitialOutput=0
  wires:
  HWT dem/1 -> If Action Subsystem1/5(HWT dem)
  EGO dis/1 -> If Action Subsystem1/4(Ego distance)
  e/1 -> If Action Subsystem1/2(e)
  If Action Subsystem/2(throttle) -> Merge1/1
  If Action Subsystem1/1(dec) -> Merge/2
  Merge1/1 -> throttle/1
  Merge/1 -> dec/1
  If Action Subsystem1/2(throttle) -> Merge1/2
  If Action Subsystem/1(dec) -> Merge/1
  Vp/1 -> If Action Subsystem1/3(Vp)
  If/2 -> If Action Subsystem1/Action
  If/1 -> If Action Subsystem/Action
  rd/1 -> If Action Subsystem1/1(rd), If/1

== system ACC_speed_change_curve_cs/Audi_A8_1/ACC_System3/TIS2 ACC action/Stop & Go ==
  Brake_Pres_in[bar] : Inport
  Throttle_in[%] : Inport  Port=2
  TIS2_Distance[m] : Inport  Port=3
  TIS2_HWT_flag : Inport  Port=4
  TIS2_Safe_Distance [m] : Inport  Port=5
  Vp [m/s] : Inport  Port=6
  Rangedot [m/s] : Inport  Port=7
  EGO_Velocity [m/s] : Inport  Port=8
  Stand : Inport  Port=9
  Gain : Gain  Gain=3.6
  If : If  IfExpression=u1 == 1
  If Action Subsystem : Subsystem  TreatAsAtomicUnit=on
  If Action Subsystem1 : Subsystem  TreatAsAtomicUnit=on
  Logical Operator : Logic  AllPortsSameDT=off  OutDataTypeStr=boolean
  LowActiv : Constant  Value=LowSpeedActv
  Merge : Merge
  Merge1 : Merge
  Rangedot [m/s]1 : InportShadow  Port=7
  Relational Operator1 : RelationalOperator  Operator=>  OutDataTypeStr=boolean
  Subsystem : Subsystem
  BrakePres[bar] : Outport
  Th_out [%] : Outport  Port=2
  wires:
  Stand/1 -> If Action Subsystem/6(Stand)
  Merge1/1 -> Subsystem/2(In2)
  Relational Operator1/1 -> Logical Operator/2
  TIS2_HWT_flag/1 -> Logical Operator/1
  If Action Subsystem/2(th) -> Merge/1
  If Action Subsystem/1(br) -> Merge1/1
  Rangedot [m/s]/1 -> If Action Subsystem/3(rd)
  EGO_Velocity [m/s]/1 -> Subsystem/3(EGO_Velocity [m/s])
  Subsystem/1(BrakePres[bar]) -> BrakePres[bar]/1
  Rangedot [m/s]1/1 -> Subsystem/1(In1)
  If Action Subsystem1/1(Out1) -> Merge/2
  If/1 -> If Action Subsystem/Action
  If Action Subsystem1/2(Out2) -> Merge1/2
  Merge/1 -> Th_out [%]/1
  Brake_Pres_in[bar]/1 -> If Action Subsystem1/2(In2)
  Throttle_in[%]/1 -> If Action Subsystem/4(th_in), If Action Subsystem1/1(In1)
  If/2 -> If Action Subsystem1/Action
  Gain/1 -> Relational Operator1/2
  Logical Operator/1 -> If/1
  LowActiv/1 -> Relational Operator1/1
  Vp [m/s]/1 -> If Action Subsystem/5(Vp), Gain/1
  TIS2_Safe_Distance [m]/1 -> If Action Subsystem/2(TIS2_Safe_Distance [m])
  TIS2_Distance[m]/1 -> If Action Subsystem/1(TIS2_Distance[m])

== system ACC_speed_change_curve_cs/Audi_A8_1/ACC_System3/TIS2 Bend Road/Hold ==
  HWTflagIN : Inport
  lead_vel_in : Inport  Port=2
  HWTflagIN1 : InportShadow
  If : If  IfExpression=u1 < 0.1  SampleTime=Tsensor
  If Action Subsystem : Subsystem  TreatAsAtomicUnit=on
  If Action Subsystem1 : Subsystem  TreatAsAtomicUnit=on
  Merge : Merge
  HWT_flag : Outport
  wires:
  HWTflagIN1/1 -> If Action Subsystem/1(In1)
  HWTflagIN/1 -> If Action Subsystem1/1(In1)
  Merge/1 -> HWT_flag/1
  If Action Subsystem1/1(Out1) -> Merge/2
  If Action Subsystem/1(Out1) -> Merge/1
  If/2 -> If Action Subsystem1/Action
  If/1 -> If Action Subsystem/Action
  lead_vel_in/1 -> If/1

== system ACC_speed_change_curve_cs/Audi_A8_1/ACC_System3/TIS2 Bend Road/Lead Car Longitudinal Velocity ==
  note: === TIS2 Lead Car Longitudinal Velocity block ===
      |
      |  - computes the leading car absolute velocity and safe distance between the EGO and leading car.
  HWT_dem (s) : Inport
  TIS1 Rangedot [m/s] : Inport  Port=2
  EGO Velocity [m/s] : Inport  Port=3
  Standstill [m] : Inport  Port=4
  theta [rad] : Inport  Port=5
  lambda [rad] : Inport  Port=6
  TIS2 Range [m] : Inport  Port=7
  Abs : Abs
  Add : Sum  Inputs=+-
  Add1 : Sum  Inputs=+-
  Constant : Constant  Value=0
  Divide : Product  Inputs=*/
  Divide2 : Product  Inputs=*/
  HWT_dem (s)1 : InportShadow
  Product : Product  RndMeth=Zero
  Relational Operator : RelationalOperator  Operator=<=  OutDataTypeStr=boolean
  Switch : Switch  Criteria=u2 > Threshold
  Switch1 : Switch  Threshold=5*TISMaxRange(2)
  Trigonometric Function : Trigonometry  Operator=cos
  Safe distance [m] : Outport
  Lead velocity [m/s] : Outport  Port=2
  wires:
  Switch1/1 -> Lead velocity [m/s]/1
  Constant/1 -> Switch1/1
  TIS2 Range [m]/1 -> Switch1/2
  Abs/1 -> Switch1/3, Relational Operator/1, Product/1
  EGO Velocity [m/s]/1 -> Add/1
  Divide2/1 -> Add/2
  Trigonometric Function/1 -> Divide2/2
  Add1/1 -> Trigonometric Function/1
  theta [rad]/1 -> Add1/2
  lambda [rad]/1 -> Add1/1
  TIS1 Rangedot [m/s]/1 -> Divide2/1
  Add/1 -> Abs/1
  HWT_dem (s)/1 -> Product/2
  Product/1 -> Switch/3
  Switch/1 -> Safe distance [m]/1
  Standstill [m]/1 -> Divide/1, Switch/1
  HWT_dem (s)1/1 -> Divide/2
  Divide/1 -> Relational Operator/2
  Relational Operator/1 -> Switch/2

== system ACC_speed_change_curve_cs/Audi_A8_1/ACC_System3/TIS2 Bend Road/TIS1 HWT Computing ==
  note: === TIS1 HWT Computing block===
      |
      |  - computes HeadWay Time (HWT) as it is defined in ISO norms.
  Distance [m] : Inport
  Velocity [m/s] : Inport  Port=2
  If : If
  If Action Subsystem : Subsystem  TreatAsAtomicUnit=on
  If Action Subsystem1 : Subsystem  TreatAsAtomicUnit=on
  Merge : Merge
  HWT [s] : Outport
  wires:
  Distance [m]/1 -> If Action Subsystem/1(Distance [m])
  Merge/1 -> HWT [s]/1
  If Action Subsystem1/1(Out1) -> Merge/2
  If Action Subsystem/1(HWT [s]) -> Merge/1
  If/2 -> If Action Subsystem1/Action
  If/1 -> If Action Subsystem/Action
  Velocity [m/s]/1 -> If Action Subsystem/2(Velocity [m/s]), If/1

== system ACC_speed_change_curve_cs/Audi_A8_1/ACC_System3/TIS2 Bend Road/TIS2 Closest Object On Bend Road ==
  note: === TIS2 Closest Object block ===
      |
      |  - passing through data about potentially the most dangerous object driving on the bend road.
  index : Inport
  TIS2_range [m] : Inport  Port=2
  TIS2_rangedot [m] : Inport  Port=3
  TIS2_theta [rad] : Inport  Port=4
  TIS2_Distance [m] : Inport  Port=5
  TIS2_lambda [rad] : Inport  Port=6
  Constant2 : Constant  Value=5*TISMaxRange(2)
  Selector{1..3,6..7} (5 alike) : Selector  InputPortWidth=TISdet(2)  IndexOptions=Index vector (port)  Indices=[1 3]  OutputSizes=1
  Switch : Switch  Criteria=u2 ~= 0
  rangedot [m/s] : Outport
  theta [rad] : Outport  Port=2
  Distance [m] : Outport  Port=3
  range [m] : Outport  Port=4
  lambda [rad] : Outport  Port=5
  wires:
  Switch/1 -> Distance [m]/1
  Constant2/1 -> Switch/3
  Selector6/1 -> Switch/1, Switch/2
  Selector7/1 -> lambda [rad]/1
  Selector3/1 -> theta [rad]/1
  Selector2/1 -> rangedot [m/s]/1
  Selector1/1 -> range [m]/1
  TIS2_lambda [rad]/1 -> Selector7/1
  TIS2_Distance [m]/1 -> Selector6/1
  TIS2_theta [rad]/1 -> Selector3/1
  index/1 -> Selector7/2, Selector6/2, Selector3/2, Selector2/2, Selector1/2
  TIS2_range [m]/1 -> Selector1/1
  TIS2_rangedot [m]/1 -> Selector2/1

== system ACC_speed_change_curve_cs/Audi_A8_1/ACC_System3/TIS2 Bend Road/TIS2 HWT Flag ==
  note: === TIS2 HWT Flag block ===
      |
      |  - outputs the HeadWay Time (HWT) flag,
      |  - holds a high level if the criteria were met,
      |  - sets HWT flag to low level if leading car
      |    went outside the scope of the sensors.
  Distance closest [m] : Inport
  HWT [s] : Inport  Port=2
  HWT_dem [s] : Inport  Port=3
  Standstill distance : Inport  Port=4
  Abs : Abs
  Compare To Constant1 : simulink/Logic and Bit Operations/Compare To Constant  relop===  const=5*TISMaxRange(2)  OutDataTypeStr=uint8
  Constant : Constant
  Constant1 : Constant  Value=0
  Data Type Conversion : DataTypeConversion
  Data Type Conversion1 : DataTypeConversion
  Discrete-Time Integrator : DiscreteIntegrator  ExternalReset=level  SampleTime=Tsensor  ICPrevOutput=DiscIntNeverNeededParam  ICPrevScaledInput=DiscIntNeverNeededParam
  Distance closest [m]1 : InportShadow
  Gain : Gain  Gain=2
  Gain1 : Gain
  Gain2 : Gain  Gain=100
  Gain3 : Gain  Gain=1e6  OutDataTypeStr=double
  Gain4 : Gain  Gain=1.25
  Gain5 : Gain  Gain=1.25
  Gain6 : Gain  Gain=0.01
  Gain7 : Gain  Gain=1e6  OutDataTypeStr=double
  HWT [s]1 : InportShadow  Port=2
  HWT [s]2 : InportShadow  Port=2
  HWT_dem [s]1 : InportShadow  Port=3
  HWT_dem [s]2 : InportShadow  Port=3
  Logical Operator : Logic  AllPortsSameDT=off  OutDataTypeStr=boolean
  Logical Operator1 : Logic  AllPortsSameDT=off  OutDataTypeStr=boolean
  Logical Operator2 : Logic  Operator=OR  Inputs=3  AllPortsSameDT=off  OutDataTypeStr=boolean
  Logical Operator3 : Logic  AllPortsSameDT=off  OutDataTypeStr=boolean
  MinMax : MinMax
  MinMax1 : MinMax
  Relational Operator : RelationalOperator  Operator=<=  OutDataTypeStr=boolean
  Relational Operator1 : RelationalOperator  OutDataTypeStr=boolean
  Relational Operator2 : RelationalOperator  Operator=>  OutDataTypeStr=boolean
  Relational Operator3 : RelationalOperator  Operator=>  OutDataTypeStr=boolean
  Rounding Function : Rounding
  Sum of Elements : Sum  Inputs=+
  Switch : Switch  Criteria=u2 > Threshold
  HWT_flag : Outport
  wires:
  Gain7/1 -> Discrete-Time Integrator/2
  Data Type Conversion1/1 -> Gain3/1
  Data Type Conversion/1 -> Gain7/1
  Relational Operator3/1 -> Logical Operator2/3
  Gain5/1 -> Relational Operator3/2
  Gain6/1 -> Relational Operator3/1
  MinMax1/1 -> Gain2/1
  Rounding Function/1 -> Gain6/1
  Gain2/1 -> Rounding Function/1
  Logical Operator2/1 -> Data Type Conversion/1
  HWT [s]2/1 -> MinMax1/1
  HWT_dem [s]2/1 -> Gain5/1
  Gain4/1 -> Relational Operator/2
  Discrete-Time Integrator/1 -> Abs/1
  Constant1/1 -> Switch/3
  Constant/1 -> Switch/1
  Abs/1 -> Switch/2
  Switch/1 -> HWT_flag/1
  Gain3/1 -> Discrete-Time Integrator/1
  Logical Operator3/1 -> Logical Operator2/2
  MinMax/1 -> Logical Operator3/1
  Relational Operator2/1 -> Logical Operator3/2
  Standstill distance/1 -> Relational Operator2/2
  Distance closest [m]1/1 -> Relational Operator2/1
  HWT_dem [s]1/1 -> Gain/1
  Gain1/1 -> MinMax/1
  Relational Operator1/1 -> Gain1/1
  Gain/1 -> Relational Operator1/2
  HWT [s]1/1 -> Relational Operator1/1
  Compare To Constant1/1 -> Logical Operator1/1, Logical Operator1/2
  HWT [s]/1 -> Relational Operator/1
  HWT_dem [s]/1 -> Gain4/1
  Relational Operator/1 -> Sum of Elements/1
  Sum of Elements/1 -> Logical Operator/1, Logical Operator/2
  Logical Operator/1 -> Data Type Conversion1/1
  Distance closest [m]/1 -> Compare To Constant1/1
  Logical Operator1/1 -> Logical Operator2/1
